simulink subsystem "Reference_Generator"  (R2024a)
settings: Solver=VariableStepAuto  StartTime=0.0  StopTime=10.0  RelTol=1e-3
undefined symbols (not defined in the file): eta_IC
libraries: vrlib x1
settings Model: Creator=esben  LastModifiedBy=BP21JL
settings SolverCC: AlgebraicLoopSolver=TrustRegion
settings DebuggingCC: UnconnectedInputMsg=warning  UnconnectedOutputMsg=warning  UnconnectedLineMsg=warning
settings ModelReferenceCC: EnableRefExpFcnMdlSchedulingChecks=on
settings RTWCC: GPUComputeCapability=3.5  DLArmComputeVersion=19.05

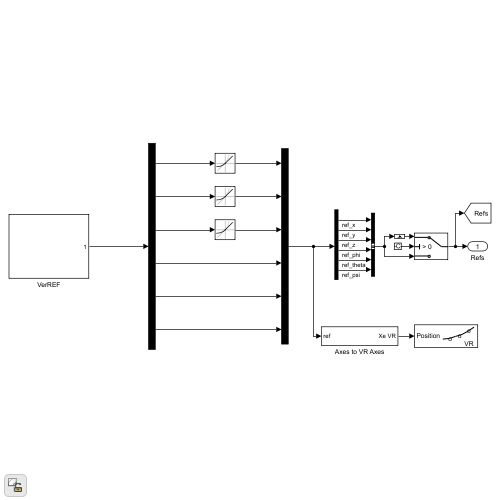
[thumbnail: Simulink's stored preview of the top-level diagram]
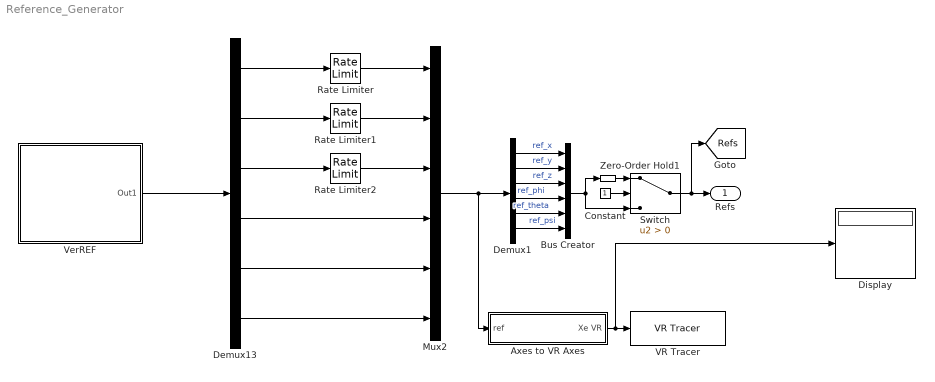
== system Reference_Generator ==
  Axes to VR Axes : Subsystem
  Bus Creator : BusCreator  Inputs=6  OutDataTypeStr=Bus: eta
      settings: InheritFromInputs=off
  Constant : Constant
  Demux1 : Demux  Outputs=6
  Demux13 : Demux  Outputs=6
  Display : Display
  Mux2 : Mux  Inputs=6
  Rate Limiter : RateLimiter  RisingSlewLimit=0.7*2  FallingSlewLimit=-0.7*2  SampleTimeMode=inherited  InitialCondition=eta_IC.N
  Rate Limiter1 : RateLimiter  RisingSlewLimit=0.5*2  FallingSlewLimit=-0.5*2  SampleTimeMode=inherited  InitialCondition=eta_IC.E
  Rate Limiter2 : RateLimiter  RisingSlewLimit=0.7*2  FallingSlewLimit=-0.7*2  SampleTimeMode=inherited  InitialCondition=eta_IC.D
  Switch : Switch  Criteria=u2 > Threshold  SaturateOnIntegerOverflow=off  InputSameDT=off
  VR Tracer : vrlib/VR Tracer  VrmlFile=C:\Users\BP21JL\AppData\Roaming\MathWorks\MATLAB Add-Ons\Apps\ROVSimulator\Dependencies\Animation\Good_world_BlueRov.x3d  MarkerName=Octahedron  UseLines=on  UseTriads=on  MarkerScale=0.02*[1 1 1]  MarkerColorSelection=Selected from color list  MarkerColor=yellow  rgbval=[0 1 1]  Ts=1  ForceViewerOpen=off  ConnectPlane=off  PlaneCoeff=[0 1 0 0]  ConnectPoint=None  PointCoord=[0 0 0]
  "VerREF " : Subsystem
  Zero-Order Hold1 : ZeroOrderHold  SampleTime=1/20
  Refs : Outport
  tag scope: Refs=global
  wires:
  Demux13/3 -> Rate Limiter2/1
  Demux13/5 -> Mux2/5
  "VerREF "/1(Out1) -> Demux13/1
  Demux13/4 -> Mux2/4
  Mux2/1 -> Axes to VR Axes/1(ref), Demux1/1
  Rate Limiter1/1 -> Mux2/2
  Rate Limiter/1 -> Mux2/1
  Demux13/2 -> Rate Limiter1/1
  Demux13/1 -> Rate Limiter/1
  Rate Limiter2/1 -> Mux2/3
  Demux1/1 -> Bus Creator/1  "ref_x"
  Demux1/2 -> Bus Creator/2  "ref_y"
  Demux1/3 -> Bus Creator/3  "ref_z"
  Demux1/4 -> Bus Creator/4  "ref_phi"
  Demux1/5 -> Bus Creator/5  "ref_theta"
  Demux1/6 -> Bus Creator/6  "ref_psi"
  Demux13/6 -> Mux2/6
  Switch/1 -> Refs/1, [Refs]
  Bus Creator/1 -> Zero-Order Hold1/1, Switch/3
  Constant/1 -> Switch/2
  Zero-Order Hold1/1 -> Switch/1
  Axes to VR Axes/1(Xe VR) -> VR Tracer/1, Display/1

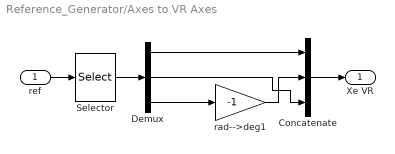
== system Reference_Generator/Axes to VR Axes ==
  ref : Inport
  Concatenate : Concatenate  NumInputs=3
  Demux : Demux  Outputs=3
      settings: DisplayOption=none
  Selector : Selector  InputPortWidth=6  IndexOptions=Index vector (dialog)  Indices=[1 2 3]  OutputSizes=1
  rad-->deg1 : Gain  Gain=-1  SaturateOnIntegerOverflow=on  OutDataTypeStr=Inherit: Same as input  ParamDataTypeStr=Inherit: Same as input
  Xe VR : Outport  VectorParamsAs1DForOutWhenUnconnected=off
  wires:
  Selector/1 -> Demux/1
  Demux/1 -> Concatenate/1
  rad-->deg1/1 -> Concatenate/2
  Concatenate/1 -> Xe VR/1
  Demux/3 -> rad-->deg1/1
  Demux/2 -> Concatenate/3
  ref/1 -> Selector/1

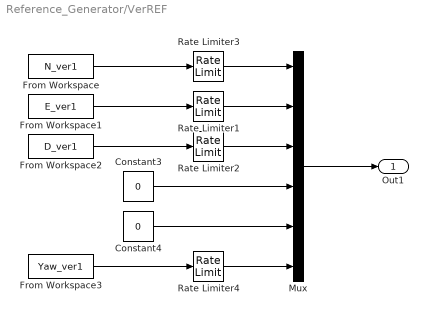
== system Reference_Generator/VerREF  ==
  Constant3 : Constant  Value=0
  Constant4 : Constant  Value=0
  From Workspace : FromWorkspace  VariableName=N_ver1  SampleTime=-1
  From Workspace1 : FromWorkspace  VariableName=E_ver1  SampleTime=-1
  From Workspace2 : FromWorkspace  VariableName=D_ver1  SampleTime=-1
  From Workspace3 : FromWorkspace  VariableName=Yaw_ver1  SampleTime=-1
  Mux : Mux  Inputs=6
  Rate Limiter1 : RateLimiter  RisingSlewLimit=.2  FallingSlewLimit=-.2  SampleTimeMode=inherited
  Rate Limiter2 : RateLimiter  RisingSlewLimit=.2  FallingSlewLimit=-.2  SampleTimeMode=inherited
  Rate Limiter3 : RateLimiter  RisingSlewLimit=.2  FallingSlewLimit=-.2  SampleTimeMode=inherited
  Rate Limiter4 : RateLimiter  RisingSlewLimit=.05  FallingSlewLimit=-.05  SampleTimeMode=inherited
  Out1 : Outport
  wires:
  Rate Limiter4/1 -> Mux/6
  From Workspace1/1 -> Rate Limiter1/1
  From Workspace/1 -> Rate Limiter3/1
  Constant3/1 -> Mux/4
  Rate Limiter3/1 -> Mux/1
  Constant4/1 -> Mux/5
  From Workspace3/1 -> Rate Limiter4/1
  Rate Limiter2/1 -> Mux/3
  Mux/1 -> Out1/1
  Rate Limiter1/1 -> Mux/2
  From Workspace2/1 -> Rate Limiter2/1
